simulink model "simulacaoMaquinaCCv2"  (R2022a)
settings: Solver=VariableStepAuto  StartTime=0.0  StopTime=3  RelTol=1e-3
libraries: simulink x2, spsControlledVoltageSourceLib x1, spsDCMachineLib x1, spsDCVoltageSourceLib x1, spspowerguiLib x1
settings Model: Creator=marcone.faria  LastModifiedBy=marcone.faria
settings SolverCC: ZeroCrossAlgorithm=Adaptive
settings DebuggingCC: IgnoredZcDiagnostic=none

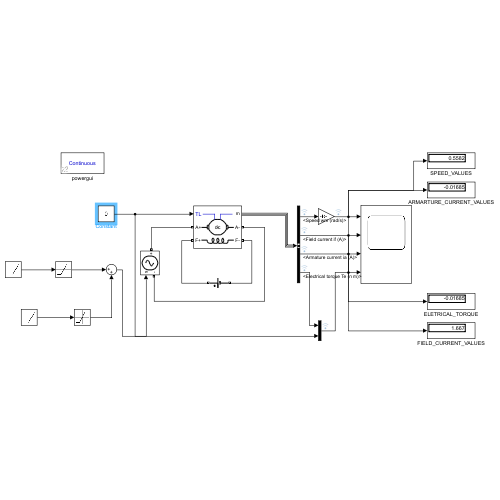
[thumbnail: Simulink's stored preview of the top-level diagram]
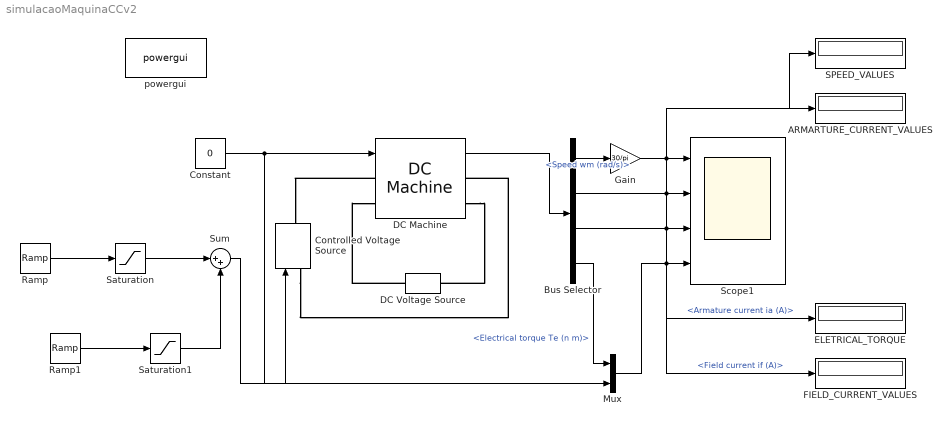
== system simulacaoMaquinaCCv2 ==
  ARMARTURE_CURRENT_VALUES : Display
  Bus Selector : BusSelector  OutputSignals=Speed wm (rad/s),Field current if (A),Armature current ia (A),Electrical torque Te (n m)
  Constant : Constant  Value=0
  Controlled Voltage Source : spsControlledVoltageSourceLib/Controlled Voltage Source  Initialize=on  Source_Type=AC  Amplitude=0  Phase=0  Frequency=0  Measurements=None
  DC Machine : spsDCMachineLib/DC Machine  PresetModel=04: 10HP 240V 1750RPM Field:300V  MechanicalLoad=Torque TL  FieldType=Wound  ShowDetailedParameters=on  MeasurementBus=off  RLa=[1.086 0.01216]  RLf=[180 71.47]  Laf=0.6458  MachineConstant=Torque constant (N.m/A)  Ke=1.8  Kt=1.8  J=0.04251  Bm=0.003406  Tf=1.046  w0=1  Ifinit=1.66666666666667  TsPowergui=0  TsBlock=-1
  DC Voltage Source : spsDCVoltageSourceLib/DC Voltage Source  Amplitude=300  Measurements=None
  ELETRICAL_TORQUE : Display
  FIELD_CURRENT_VALUES : Display
  Gain : Gain  Gain=30/pi
  Mux : Mux  Inputs=2
  Ramp : simulink/Sources/Ramp  slope=1000  start=0  InitialOutput=0
  Ramp1 : simulink/Sources/Ramp  slope=-1000  start=1.5  InitialOutput=0
  SPEED_VALUES : Display
  Saturation : Saturate  UpperLimit=240  LowerLimit=0
  Saturation1 : Saturate  UpperLimit=0  LowerLimit=-240
  Scope1 : Scope  NumInputPorts=4
  Sum : Sum  Inputs=|++
  powergui : spspowerguiLib/powergui  Priority=1  SimulationMode=Continuous  SampleTime=50e-6  frequency=60  Iterations=50  frequencyindice=0  Pbase=100e6  ErrMax=1e-4  UnitsV=kV  UnitsW=MW  buscounter=0  FunctionMessages=off  echomessages=off  EnableUseOfTLC=off  CurrentSourceSwitches=off  DisableSnubberDevices=off  DisableRonSwitches=off  DisableVfSwitches=off  DisplayEquations=off  AutomaticDiscreteSolvers=off  SolverType=Tustin/Backward Euler (TBE)  Interpol=off  ExternalGateDelay=off  methode=off  Ts=100  x0status=blocks  SPID=on  SwTol=0  HookPort=off  NonlinearTolerance=1e-4  nMaxIteration=100  ContinueOnMaxIteration=off  RestoreLinks=warning  ResistiveCurrentMeasurement=off  Frange=[0:2:500]  Ylog=off  Xlog=on  ShowGrid=off  save=off  variable=ZData  structure=0  ZoomFFT=off  StartTime=0.0  cycles=1  DisplayStyle=1  fundamental=60  FreqAxis=off  MaxFrequency=1000  frequencyindicesteady=1  RmsSteady=1  display=off
  wires:
  DC Machine/1 -> Bus Selector/1
  Constant/1 -> DC Machine/1, Mux/2
  Bus Selector/1 -> Gain/1  "<Speed wm (rad/s)>"
  Bus Selector/3 -> ARMARTURE_CURRENT_VALUES/1, Scope1/2, ELETRICAL_TORQUE/1  "<Armature current ia (A)>"
  Bus Selector/2 -> Scope1/4, FIELD_CURRENT_VALUES/1  "<Field current if (A)>"
  Gain/1 -> Scope1/1, SPEED_VALUES/1
  Bus Selector/4 -> Mux/1  "<Electrical torque Te (n m)>"
  Mux/1 -> Scope1/3
  Sum/1 -> Controlled Voltage Source/1
  Ramp/1 -> Saturation/1
  Saturation/1 -> Sum/1
  Ramp1/1 -> Saturation1/1
  Saturation1/1 -> Sum/2
  connections:
  Controlled Voltage Source/LConn1 -- DC Machine/RConn1
  DC Machine/LConn1 -- Controlled Voltage Source/RConn1
  DC Voltage Source/RConn1 -- DC Machine/LConn2
  DC Machine/RConn2 -- DC Voltage Source/LConn1
